simulink model "Sensors"  (R2017b)
settings: Solver=FixedStepAuto  StartTime=0.0  StopTime=10.0  RelTol=1e-3
settings Model: Creator=cspt  LastModifiedBy=joser
settings RTWCC: SystemTargetFile=irt.tlc  TemplateMakefile=irt_default_tmf  Description=INTECRIO Real-Time Target
settings STFCustomTargetCC: TargetLangStandard=C99 (ISO)  UtilityFuncGeneration=Shared location  SystemTargetFile=irt.tlc
settings GRTTargetCC: UtilityFuncGeneration=Shared location  ParMdlRefBuildCompliant=off  CompOptLevelCompliant=off  ConcurrentExecutionCompliant=off  CombineOutputUpdateFcns=off  MatFileLogging=off  CPPClassGenCompliant=off  GRTInterface=on  UseToolchainInfoCompliant=off  GenerateASAP2=on

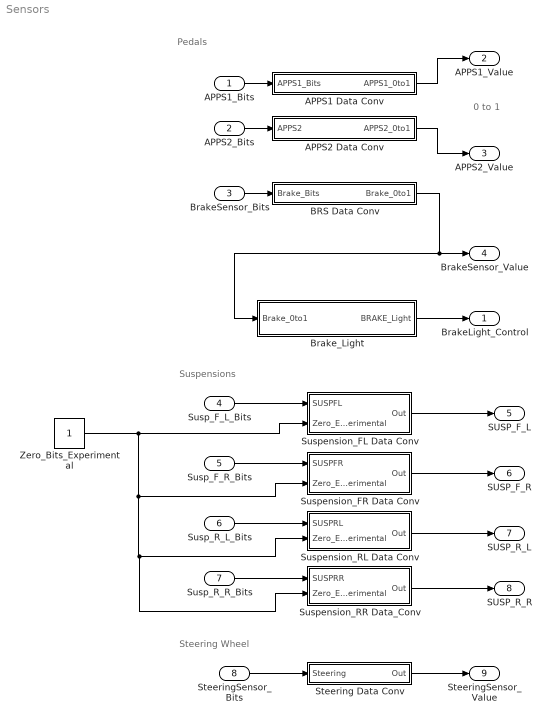
== system Sensors ==
  note: 0 to 1
  note: Pedals
  note: Suspensions
  note: Steering Wheel
  APPS1_Bits : Inport
  APPS2_Bits : Inport  Port=2
  BrakeSensor_Bits : Inport  Port=3
  Susp_F_L_Bits : Inport  Port=4
  Susp_F_R_Bits : Inport  Port=5
  Susp_R_L_Bits : Inport  Port=6
  Susp_R_R_Bits : Inport  Port=7
  SteeringSensor_Bits : Inport  Port=8
  APPS1 Data Conv : Subsystem
  "APPS2 Data Conv " : Subsystem
  BRS Data Conv : Subsystem
  Brake_Light : Subsystem  TreatAsAtomicUnit=on
  Steering Data Conv : Subsystem
  Suspension_FL Data Conv : Subsystem
  Suspension_FR Data Conv : Subsystem
  Suspension_RL Data Conv : Subsystem
  Suspension_RR Data_Conv : Subsystem
  Zero_Bits_Experimental : Constant
  BrakeLight_Control : Outport
  APPS1_Value : Outport  Port=2
  APPS2_Value : Outport  Port=3
  BrakeSensor_Value : Outport  Port=4
  SUSP_F_L : Outport  Port=5
  SUSP_F_R : Outport  Port=6
  SUSP_R_L : Outport  Port=7
  SUSP_R_R : Outport  Port=8
  SteeringSensor_Value : Outport  Port=9
  wires:
  APPS1 Data Conv/1(APPS1_0to1) -> APPS1_Value/1
  APPS1_Bits/1 -> APPS1 Data Conv/1(APPS1_Bits)
  BrakeSensor_Bits/1 -> BRS Data Conv/1(Brake_Bits)
  Brake_Light/1(BRAKE_Light) -> BrakeLight_Control/1
  BRS Data Conv/1(Brake_0to1) -> BrakeSensor_Value/1, Brake_Light/1(Brake_0to1)
  "APPS2 Data Conv "/1(APPS2_0to1) -> APPS2_Value/1
  APPS2_Bits/1 -> "APPS2 Data Conv "/1(APPS2)
  Susp_F_R_Bits/1 -> Suspension_FR Data Conv/1(SUSPFR)
  Susp_R_R_Bits/1 -> Suspension_RR Data_Conv/1(SUSPRR)
  Susp_R_L_Bits/1 -> Suspension_RL Data Conv/1(SUSPRL)
  Susp_F_L_Bits/1 -> Suspension_FL Data Conv/1(SUSPFL)
  Suspension_FL Data Conv/1(Out) -> SUSP_F_L/1
  Suspension_RR Data_Conv/1(Out) -> SUSP_R_R/1
  Suspension_FR Data Conv/1(Out) -> SUSP_F_R/1
  Suspension_RL Data Conv/1(Out) -> SUSP_R_L/1
  Zero_Bits_Experimental/1 -> Suspension_RR Data_Conv/2(Zero_Experimental), Suspension_RL Data Conv/2(Zero_Experimental), Suspension_FR Data Conv/2(Zero_Experimental), Suspension_FL Data Conv/2(Zero_Experimental)
  SteeringSensor_Bits/1 -> Steering Data Conv/1("Steering ")
  Steering Data Conv/1(Out) -> SteeringSensor_Value/1

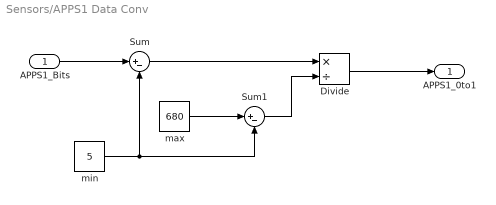
== system Sensors/APPS1 Data Conv ==
  APPS1_Bits : Inport
  Divide : Product  Inputs=*/
  Sum : Sum  Inputs=|+-
  Sum1 : Sum  Inputs=|+-
  max : Constant  Value=680
  min : Constant  Value=5
  APPS1_0to1 : Outport
  wires:
  APPS1_Bits/1 -> Sum/1
  min/1 -> Sum/2, Sum1/2
  max/1 -> Sum1/1
  Sum/1 -> Divide/1
  Sum1/1 -> Divide/2
  Divide/1 -> APPS1_0to1/1

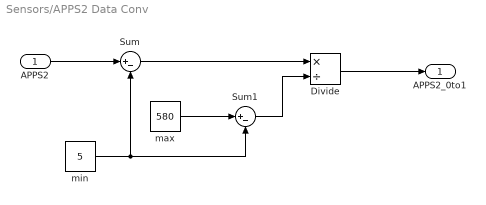
== system Sensors/APPS2 Data Conv  ==
  APPS2 : Inport
  Divide : Product  Inputs=*/
  Sum : Sum  Inputs=|+-
  Sum1 : Sum  Inputs=|+-
  max : Constant  Value=580
  min : Constant  Value=5
  APPS2_0to1 : Outport
  wires:
  APPS2/1 -> Sum/1
  min/1 -> Sum/2, Sum1/2
  max/1 -> Sum1/1
  Sum/1 -> Divide/1
  Sum1/1 -> Divide/2
  Divide/1 -> APPS2_0to1/1

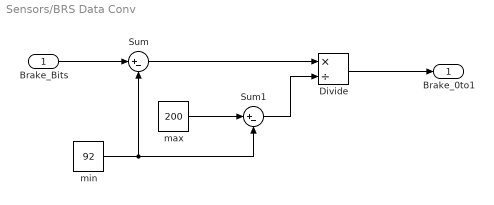
== system Sensors/BRS Data Conv ==
  Brake_Bits : Inport
  Divide : Product  Inputs=*/
  Sum : Sum  Inputs=|+-
  Sum1 : Sum  Inputs=|+-
  max : Constant  Value=200
  min : Constant  Value=92
  Brake_0to1 : Outport
  wires:
  Brake_Bits/1 -> Sum/1
  min/1 -> Sum/2, Sum1/2
  max/1 -> Sum1/1
  Sum/1 -> Divide/1
  Sum1/1 -> Divide/2
  Divide/1 -> Brake_0to1/1

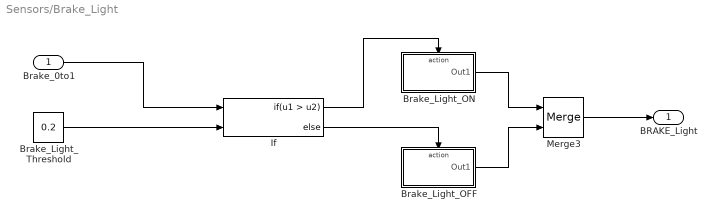
== system Sensors/Brake_Light ==
  Brake_0to1 : Inport
  Brake_Light_OFF : Subsystem  TreatAsAtomicUnit=on
  Brake_Light_ON : Subsystem  TreatAsAtomicUnit=on
  Brake_Light_Threshold : Constant  Value=0.2
  If : If  NumInputs=2  IfExpression=u1 > u2
  Merge3 : Merge
  BRAKE_Light : Outport
  wires:
  Brake_Light_Threshold/1 -> If/2
  If/1 -> Brake_Light_ON/Action
  If/2 -> Brake_Light_OFF/Action
  Brake_Light_ON/1(Out1) -> Merge3/1
  Brake_Light_OFF/1(Out1) -> Merge3/2
  Merge3/1 -> BRAKE_Light/1
  Brake_0to1/1 -> If/1

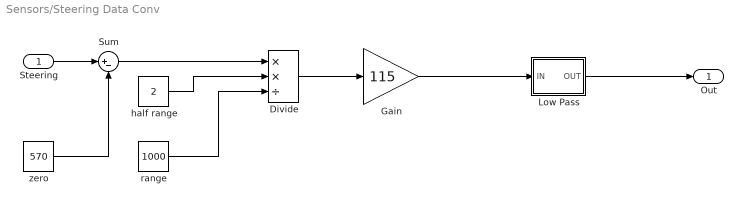
== system Sensors/Steering Data Conv ==
  "Steering " : Inport
  Divide : Product  Inputs=**/
  Gain : Gain  Gain=115
  Low Pass : Subsystem  TreatAsAtomicUnit=on
  Sum : Sum  Inputs=|+-
  half range : Constant  Value=2
  range : Constant  Value=1000
  zero : Constant  Value=570
  Out : Outport
  wires:
  zero/1 -> Sum/2
  Sum/1 -> Divide/1
  Divide/1 -> Gain/1
  range/1 -> Divide/3
  half range/1 -> Divide/2
  "Steering "/1 -> Sum/1
  Gain/1 -> Low Pass/1(IN)
  Low Pass/1(OUT) -> Out/1

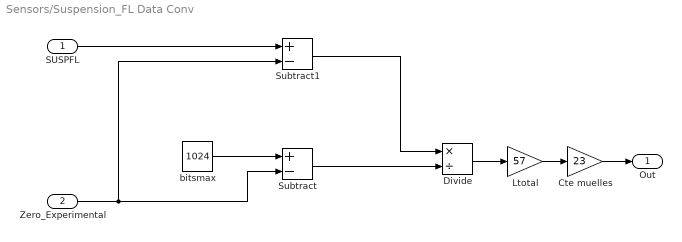
== system Sensors/Suspension_FL Data Conv ==
  SUSPFL : Inport
  Zero_Experimental : Inport  Port=2
  Cte muelles : Gain  Gain=23
  Divide : Product  Inputs=*/
  Ltotal : Gain  Gain=57
  Subtract : Sum  Inputs=+-
  Subtract1 : Sum  Inputs=+-
  "bitsmax " : Constant  Value=1024
  Out : Outport
  wires:
  Divide/1 -> Ltotal/1
  Cte muelles/1 -> Out/1
  Ltotal/1 -> Cte muelles/1
  SUSPFL/1 -> Subtract1/1
  "bitsmax "/1 -> Subtract/1
  Subtract/1 -> Divide/2
  Subtract1/1 -> Divide/1
  Zero_Experimental/1 -> Subtract1/2, Subtract/2

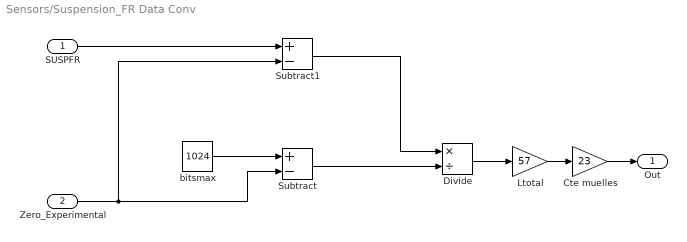
== system Sensors/Suspension_FR Data Conv ==
  SUSPFR : Inport
  Zero_Experimental : Inport  Port=2
  Cte muelles : Gain  Gain=23
  Divide : Product  Inputs=*/
  Ltotal : Gain  Gain=57
  Subtract : Sum  Inputs=+-
  Subtract1 : Sum  Inputs=+-
  "bitsmax " : Constant  Value=1024
  Out : Outport
  wires:
  Divide/1 -> Ltotal/1
  Cte muelles/1 -> Out/1
  Ltotal/1 -> Cte muelles/1
  Zero_Experimental/1 -> Subtract1/2, Subtract/2
  SUSPFR/1 -> Subtract1/1
  Subtract1/1 -> Divide/1
  Subtract/1 -> Divide/2
  "bitsmax "/1 -> Subtract/1

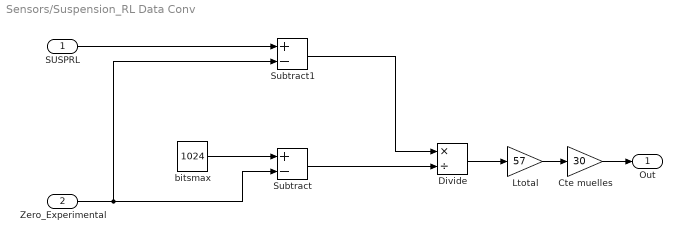
== system Sensors/Suspension_RL Data Conv ==
  SUSPRL : Inport
  Zero_Experimental : Inport  Port=2
  Cte muelles : Gain  Gain=30
  Divide : Product  Inputs=*/
  Ltotal : Gain  Gain=57
  Subtract : Sum  Inputs=+-
  Subtract1 : Sum  Inputs=+-
  "bitsmax " : Constant  Value=1024
  Out : Outport
  wires:
  Cte muelles/1 -> Out/1
  Ltotal/1 -> Cte muelles/1
  Divide/1 -> Ltotal/1
  Zero_Experimental/1 -> Subtract1/2, Subtract/2
  Subtract1/1 -> Divide/1
  "bitsmax "/1 -> Subtract/1
  Subtract/1 -> Divide/2
  SUSPRL/1 -> Subtract1/1

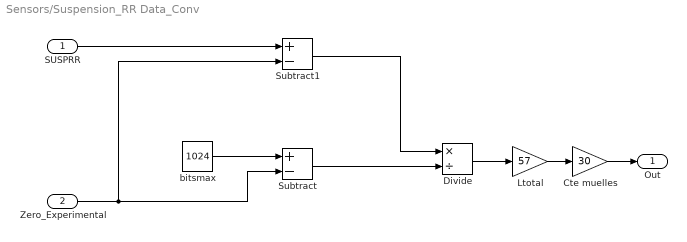
== system Sensors/Suspension_RR Data_Conv ==
  SUSPRR : Inport
  Zero_Experimental : Inport  Port=2
  Cte muelles : Gain  Gain=30
  Divide : Product  Inputs=*/
  Ltotal : Gain  Gain=57
  Subtract : Sum  Inputs=+-
  Subtract1 : Sum  Inputs=+-
  "bitsmax " : Constant  Value=1024
  Out : Outport
  wires:
  Cte muelles/1 -> Out/1
  Ltotal/1 -> Cte muelles/1
  Divide/1 -> Ltotal/1
  Zero_Experimental/1 -> Subtract1/2, Subtract/2
  Subtract1/1 -> Divide/1
  "bitsmax "/1 -> Subtract/1
  Subtract/1 -> Divide/2
  SUSPRR/1 -> Subtract1/1

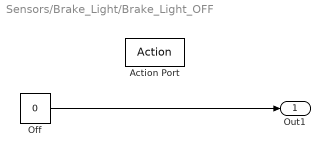
== system Sensors/Brake_Light/Brake_Light_OFF ==
  Action Port : ActionPort  ActionType=else
  Off : Constant  Value=0
  Out1 : Outport
  wires:
  Off/1 -> Out1/1

== system Sensors/Brake_Light/Brake_Light_ON ==
  Action Port : ActionPort  ActionType=then
  ON : Constant
  Out1 : Outport
  wires:
  ON/1 -> Out1/1

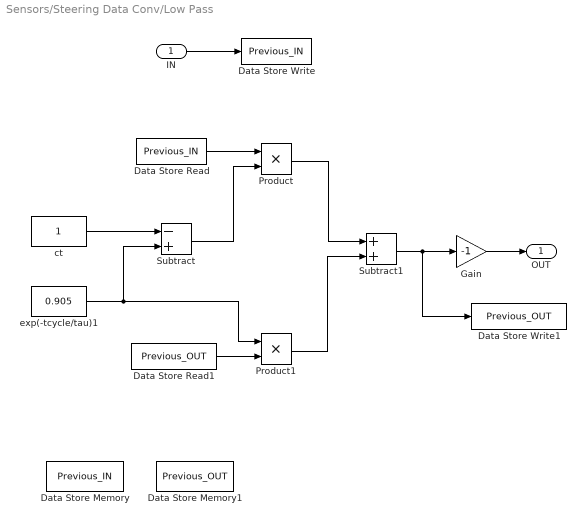
== system Sensors/Steering Data Conv/Low Pass ==
  IN : Inport
  Data Store Memory : DataStoreMemory  DataStoreName=Previous_IN  ReadBeforeWriteMsg=warning  WriteAfterWriteMsg=warning  WriteAfterReadMsg=warning  ShowAdditionalParam=off
  Data Store Memory1 : DataStoreMemory  DataStoreName=Previous_OUT  ReadBeforeWriteMsg=warning  WriteAfterWriteMsg=warning  WriteAfterReadMsg=warning  ShowAdditionalParam=off
  Data Store Read : DataStoreRead  DataStoreName=Previous_IN
  Data Store Read1 : DataStoreRead  DataStoreName=Previous_OUT
  Data Store Write : DataStoreWrite  DataStoreName=Previous_IN
  Data Store Write1 : DataStoreWrite  DataStoreName=Previous_OUT
  Gain : Gain  Gain=-1
  Product : Product
  Product1 : Product
  Subtract : Sum  Inputs=-+
  Subtract1 : Sum
  ct : Constant
  exp(-tcycle/tau)1 : Constant  Value=0.905
  OUT : Outport
  wires:
  IN/1 -> Data Store Write/1
  Data Store Read/1 -> Product/1
  Data Store Read1/1 -> Product1/2
  ct/1 -> Subtract/1
  Subtract/1 -> Product/2
  exp(-tcycle/tau)1/1 -> Product1/1, Subtract/2
  Product/1 -> Subtract1/1
  Product1/1 -> Subtract1/2
  Subtract1/1 -> Gain/1, Data Store Write1/1
  Gain/1 -> OUT/1
